simulink model "homing_ldm_aggiornat"  (R2017a)
settings: Solver=FixedStepAuto  StartTime=0.0  StopTime=inf  FixedStep=1e-3  RelTol=1e-3  EnableMultiTasking=on
values from neighbouring files (symbols this model uses):
  Acc_asse_x = []    [main_Strategia_di_pilotaggio.m]
  Acc_asse_y = []    [main_Strategia_di_pilotaggio.m]
  ppx_c = pos_poli_cc_x(mx, acx, 2)    [main_Strategia_di_pilotaggio.m]
  ppy_c = pos_poli_cc_y(my, acy, 2)    [main_Strategia_di_pilotaggio.m]
  time = 0:tf/np:tf    [Main_traiettoria.m]    (also in Main_traiettoria_ordinato.m = 0:passo:tsim)
  Vel_asse_x = []    [main_Strategia_di_pilotaggio.m]
  Vel_asse_y = []    [main_Strategia_di_pilotaggio.m]
  x = zeros(length(time),1)    [Main_traiettoria.m]    (also in Main_traiettoria_ordinato.m; main_Strategia_di_pilotaggio.m = [])
  y = zeros(length(time),1)    [Main_traiettoria.m]    (also in Main_traiettoria_ordinato.m; main_Strategia_di_pilotaggio.m = [])
undefined symbols (not defined in the file or in its folder): parx, pary, x_ref
libraries: xpcnilib x10, simulink x5
settings Model: SimulationMode=external  Creator=Davide  LastModifiedBy=stefa
settings SolverCC: EnableConcurrentExecution=on  ConcurrentTasks=on  AutoInsertRateTranBlk=on
settings DataIOCC: SaveFormat=StructureWithTime
settings OptimizationCC: BlockReduction=off  OptimizeBlockIOStorage=off  BufferReuse=off  GlobalBufferReuse=off  ExpressionFolding=off  LocalBlockOutputs=off
settings HardwareCC: ProdBitPerPointer=32  ProdBitPerSizeT=32  ProdBitPerPtrDiffT=32  ProdLargestAtomicFloat=None  ProdWordSize=32  ProdLongLongMode=on  ProdHWDeviceType=Generic->32-bit x86 compatible
settings RTWCC: SystemTargetFile=slrt.tlc  TemplateMakefile=slrt_default_tmf  Description=Simulink Real-Time  RTWCompilerOptimization=on
settings SimulinkRealTimeCC: xPCConcurrentTasks=on

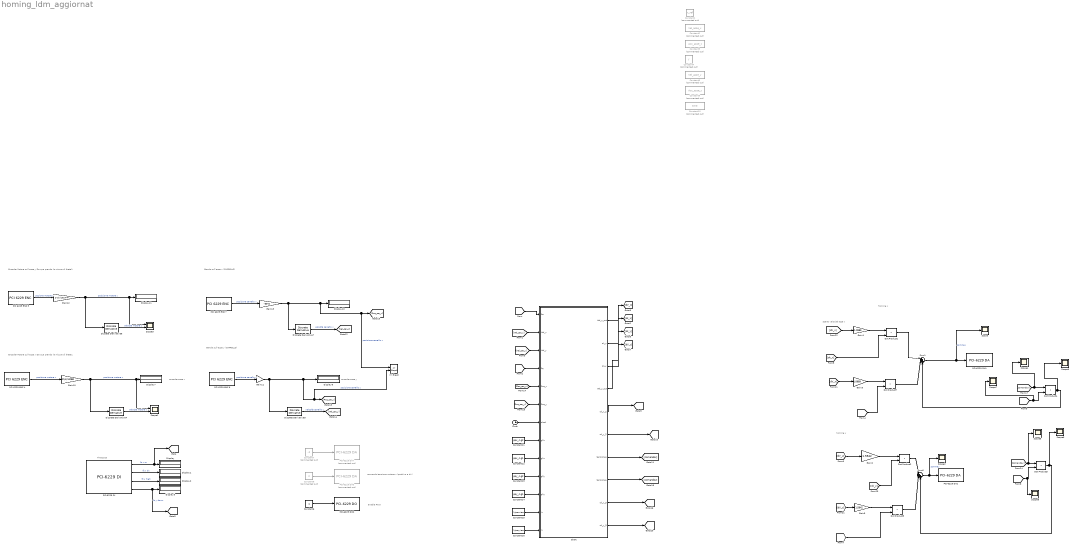
== system homing_ldm_aggiornat ==
  note: Finecorsa
  note: Encoder Motore sull'asse y
      | Da qua prendo la misura di theta1
  note: encoder asse y
  note: encoder asse x
  note: Banda sull'asse y (CARRELLO)
  note: comando tensione motore x (positivo a dx)
  note: Encoder Motore sull'asse x
      | Da qua prendo la misura di theta1
  note: enable P0.0
  note: Banda sull'asse x (CARRELLO)
  note: Scarto velocità asse x
  note: Homing x
  note: homing y
  Chart : Stateflow chart  TreatAsAtomicUnit=on
  Clock : Clock
  Constant1 : Constant  Commented=on  Value=x_ref
  Constant10 : Constant  Commented=on  Value=time
  Constant11 : Constant  Value=ppx_c.g2
  Constant12 : Constant  Value=ppx_c.g1
  Constant13 : Constant  Value=ppy_c.g2
  Constant14 : Constant  Value=ppy_c.g1
  Constant15 : Constant  Value=1/parx.tau
  Constant16 : Constant  Value=1/pary.tau
  Constant2 : Constant  Commented=on  Value=Vel_asse_x
  Constant3 : Constant  Commented=on  Value=Acc_asse_x
  Constant4 : Constant  Commented=on  Value=y
  Constant5 : Constant  Commented=on  Value=Vel_asse_y
  Constant6 : Constant
  Constant7 : Constant  Commented=on  Value=-2
  Constant8 : Constant  Commented=on  Value=2
  Constant9 : Constant  Commented=on  Value=Acc_asse_y
  Discrete Derivative{4..7} (4 alike) : simulink/Discrete/Discrete Derivative  gainval=1.0  ICPrevScaledInput=0.0  OutMin=[]  OutMax=[]  OutDataType=fixdt(1, 16)  OutScaling=2^-10  DoSatur=off
  Display{,1..3,7..8,10..11} (8 alike) : Display
  Dot Product{1..4,7..8} (6 alike) : DotProduct  InputSameDT=on  OutDataTypeStr=Inherit: Inherit via internal rule
  Gain1 : Gain  Gain=1.0989
  Gain10 : Gain  Gain=2*pi/(4096)
  Gain11 : Gain  Gain=-5e-6
  Gain12 : Gain  Gain=2*pi/(1024*4)
  Gain13 : Gain  Gain=-5e-6
  Gain2 : Gain  Gain=1.5942
  Gain3 : Gain  Gain=1.0989
  Gain5 : Gain  Gain=1.5942
  PCI 6229 ENC 4 : xpcnilib/Incremental Encoder/PCI 6229 ENC   channel=0  countMode=Quadrature Mode x4  initCount=0  reload=on  indexPhase=A low B low  filter=None  sampleTime=0.001  slot=[4 12]
      settings: SourceProductName=Simulink Real-Time  SourceProductBaseCode=XP
  PCI 6229 ENC 5 : xpcnilib/Incremental Encoder/PCI 6229 ENC   channel=1  countMode=Quadrature Mode x4  initCount=0  reload=on  indexPhase=A low B low  filter=None  sampleTime=0.001  slot=[4 12]
      settings: SourceProductName=Simulink Real-Time  SourceProductBaseCode=XP
  PCI 6229 ENC 6 : xpcnilib/Incremental Encoder/PCI 6229 ENC   channel=0  countMode=Quadrature Mode x4  initCount=0  reload=on  indexPhase=A low B low  filter=None  sampleTime=0.001  slot=[4 15]
      settings: SourceProductName=Simulink Real-Time  SourceProductBaseCode=XP
  PCI 6229 ENC 7 : xpcnilib/Incremental Encoder/PCI 6229 ENC   channel=1  countMode=Quadrature Mode x4  initCount=0  reload=on  indexPhase=A low B low  filter=None  sampleTime=0.001  slot=[4 15]
      settings: SourceProductName=Simulink Real-Time  SourceProductBaseCode=XP
  PCI-6229 DA1 : xpcnilib/D//A/M Series/PCI-6229 DA  channel=[1]  reset=[1]  initValue=[0]  sampletime=0.001  slot=[4 12]
      settings: SourceProductName=Simulink Real-Time  SourceProductBaseCode=XP
  PCI-6229 DA2 : xpcnilib/D//A/M Series/PCI-6229 DA  channel=[1]  reset=[1]  initValue=[0]  sampletime=0.001  slot=[4 15]
      settings: SourceProductName=Simulink Real-Time  SourceProductBaseCode=XP
  PCI-6229 DA6 : xpcnilib/D//A/M Series/PCI-6229 DA  Commented=on  channel=[1]  reset=[1]  initValue=[0]  sampletime=0.001  slot=[4 12]
      settings: SourceProductName=Simulink Real-Time  SourceProductBaseCode=XP
  PCI-6229 DA7 : xpcnilib/D//A/M Series/PCI-6229 DA  Commented=on  channel=[1]  reset=[1]  initValue=[0]  sampletime=0.001  slot=[4 15]
      settings: SourceProductName=Simulink Real-Time  SourceProductBaseCode=XP
  PCI-6229 DI : xpcnilib/Digital Input/M Series/PCI-6229 DI  channel=[4 5 6 7]  sampletime=0.001  slot=[4 12]
      settings: SourceProductName=Simulink Real-Time  SourceProductBaseCode=XP
  PCI-6229 DO2 : xpcnilib/Digital Output/M Series/PCI-6229 DO  channel=[1]  reset=[1]  initValue=[0]  sampletime=0.001  slot=[4 12]
      settings: SourceProductName=Simulink Real-Time  SourceProductBaseCode=XP
  Scope{,2,4..9} (8 alike) : Scope
  Scope1 : Scope  NumInputPorts=2
  Scope3 : Scope  NumInputPorts=2
  Sum1 : Sum  Inputs=|+++
  Sum6 : Sum  Inputs=|+++
  XY Graph : simulink/Sinks/XY Graph  xmin=-1  xmax=1  ymin=-1  ymax=1  st=-1
  wires:
  PCI-6229 DI/1 -> [Fcx_sx], Display/1  "fc x sx"
  PCI-6229 DI/2 -> Display1/1  "fc x dx"
  PCI-6229 DI/3 -> Display2/1  "fc y high"
  PCI-6229 DI/4 -> [Fcy_dw], Display3/1  "fc y down"
  [Fcx_sx] -> Chart/1(fcx)
  [Vel_car_x] -> Chart/2(Vel_x)
  Chart/1(Vel_x_out) -> [dV_x]
  [Fcy_dw] -> Chart/4(fcy)
  [Vel_car_y] -> Chart/3(Vel_y)
  Chart/2(ok_x) -> [ok_x]
  Chart/3(ok_y) -> [ok_y]
  Chart/4(Vel_y_out) -> [dV_y]
  [Pos_car_x] -> Chart/5(Pos_x)
  Chart/5(ok_x_2) -> [ok_x_2]
  Chart/6(ok_y_2) -> [ok_y_2]
  [Pos_car_y] -> Chart/6(Pos_y)
  Clock/1 -> Chart/7(clock)
  Gain13/1 -> Discrete Derivative7/1, XY Graph/1, [Pos_car_x], Display10/1  "posizione carrello x"
  Constant6/1 -> PCI-6229 DO2/1
  Constant8/1 -> PCI-6229 DA6/1
  Discrete Derivative4/1 -> Scope1/2  "velocità motore x"
  Discrete Derivative6/1 -> Scope3/2  "velocità motore y"
  Constant7/1 -> PCI-6229 DA7/1
  PCI 6229 ENC 5/1 -> Gain12/1  "pozione motore y"
  Discrete Derivative7/1 -> [Vel_car_x]  "velocità carrello x"
  Gain11/1 -> XY Graph/2, [Pos_car_y], Display8/1, Discrete Derivative5/1  "posizione carrello y"
  Gain10/1 -> Display7/1, Scope1/1, Discrete Derivative4/1  "posizione motore x"
  Discrete Derivative5/1 -> [Vel_car_y]  "velocità carrello y"
  PCI 6229 ENC 4/1 -> Gain10/1  "posizione motore x"
  PCI 6229 ENC 6/1 -> Gain11/1  "posizione carrello y"
  PCI 6229 ENC 7/1 -> Gain13/1  "posizione carrello x"
  Gain12/1 -> Scope3/1, Display11/1, Discrete Derivative6/1  "posizione motore y"
  Dot Product2/1 -> Sum6/1
  [dV_y] -> Gain5/1
  Gain3/1 -> Dot Product7/1
  Dot Product8/1 -> Sum6/2
  Sum6/1 -> Scope2/1, PCI-6229 DA2/1  "sommay"
  Sum1/1 -> Scope/1, PCI-6229 DA1/1  "sommax"
  Dot Product1/1 -> Sum1/1
  Gain5/1 -> Dot Product8/1
  Gain2/1 -> Dot Product2/1
  [ok_y_2] -> Dot Product8/2
  [ok_x_2] -> Dot Product7/2
  [dV_x] -> Gain3/1
  [ok_x] -> Dot Product1/2
  Dot Product7/1 -> Sum1/2
  Gain1/1 -> Dot Product1/1
  [dV_y] -> Gain2/1
  [dV_x] -> Gain1/1
  [ok_y] -> Dot Product2/2
  Constant11/1 -> Chart/8(g2x)
  Constant12/1 -> Chart/9(g1x)
  Constant13/1 -> Chart/10(g2y)
  Constant14/1 -> Chart/11(g1y)
  Constant15/1 -> Chart/12(ix)
  Constant16/1 -> Chart/13(iy)
  Chart/7(tensionex) -> [comandox]
  Chart/8(tensioney) -> [comandoy]
  Chart/10(ok_y_3) -> [ok_y_3]
  Chart/9(ok_x_3) -> [ok_x_3]
  Dot Product3/1 -> Scope6/1, Sum6/3
  [comandoy] -> Scope5/1, Dot Product3/1
  [ok_y_3] -> Scope8/1, Dot Product3/2
  Dot Product4/1 -> Scope9/1, Sum1/3
  [comandox] -> Scope4/1, Dot Product4/1
  [ok_x_3] -> Scope7/1, Dot Product4/2

== stateflow chart homing_ldm_aggiornat/Chart ==
  state Pilotaggio
    state Pilotaggio
      entry:
      t1=clock;
      ok_y_3=1;
      ok_x_3=1;
      deltax = 0;
      deltay = 0;
      deltaxp = 0;
      deltayp = 0;
      appoggio=1;
      rif_iniziale=0;
      during:
      t=clock-t1;
      if(clock-t1 ==0)
      rif_iniziale= t;
      end
      [rifx,rifxp,rify,rifyp]= interpolazione_tempi2(x, Vel_asse_x,y,Vel_asse_y,t,time,rif_iniziale)
      %[rifx,rifxp,rify,rifyp]= interpolazione_tempi2(x_i,xp_i,y_i,yp_i,u,t_m)
      deltax = Pos_x-rifx;
      deltay = Pos_y-rify;
      deltaxp = Vel_x-rifxp;
      deltayp = Vel_y-rifyp;
      %controllore posizionamento poli
      tensionex=ix*(-deltaxp*g2x-deltax*g1x)/30; %25
      tensioney=iy*(-deltayp*g2y-deltay*g1y)/50; %30
      if(tensioney>1.4)
      tensioney=1.4;
      end
      if(tensioney<-1.4)
      tensioney=-1.4;
      end
      if(tensionex>2.2)
      tensionex=2.2;
      end
      if(tensionex<-2.2)
      tensionex=-2.2;
      end
      %if tensionex ==0 && t<100
      % tensionex=2.1;
      % tensioney=0;
      % appoggio =0;
      %end
    state Fine
      entry:
      ok_y=0;
      ok_x=0;
      ok_y_2=0;
      ok_x_2=0;
      ok_y_3=0;
      ok_x_3=0;
    (default) -> Pilotaggio.Pilotaggio
    Pilotaggio.Pilotaggio -> Pilotaggio.Fine : [ abs(tensionex)==10 || abs(tensioney)==10]
  state Homing1
    state Homing_x
      entry:
      v_sp_x=-2.1;
      v_sp_y=1.2;
      ok_x=1;
      ok_y=1;
      ok_x_2=0;
      during:
      Vel_x_out = v_sp_x-Vel_x;
      Vel_y_out=v_sp_y-Vel_y;
    note: Inizializzazione asse x
        | Inizializzazione asse y
    state Fine_homing1
      entry:
      ok_y=0;
      ok_x=0;
      bx=Pos_x;
      by=Pos_y;
      v_sp_x=2.1;
      v_sp_y=-1.2;
      ok_x_2=1;
      ok_y_2=1;
      during:
      Vel_x_out=v_sp_x-Vel_x;
      dx=Pos_x-bx
      if (dx>0.6 )
      Vel_x_out=0;
      end
      Vel_y_out=v_sp_y-Vel_y;
      dy=abs(Pos_y-by);
      if (dy>0.4 )
      Vel_y_out=0;
      end
    note: Fine inizializzazione
    note: Porto al centro asse x
        | Porto al centro asse y
    state Fine
      entry:
      ok_y_2=0;
      ok_x_2=0;
      inizio_traiettoria=0;
      during:
      inizio_traiettoria=1;
    (default) -> Homing_x
    Homing_x -> Fine_homing1 : [fcx==0 && fcy==0]
    Fine_homing1 -> Homing1.Fine : [dx>0.6 && dy>0.4]
  (default) -> Homing1
  Homing1 -> Pilotaggio : [inizio_traiettoria==1]
  data: x_i function_input; xp_i function_input; y_i function_input; yp_i function_input; u function_input; t_m function_input; xx function_output; xxp function_output; yy function_output; yyp function_output; riff_iniziale function_input; t1 local double; t local double; fcx input; Vel_x_out output; Vel_x input; ok_x output; ok_y output; Vel_y input; Vel_y_out output; fcy input; Pos_x input; dx local; ok_x_2 output; v_sp_x local; v_sp_y local; Pos_y input; ok_y_2 output; dy local; clock input; bx local; by local; inizio_traiettoria local; g2x input; g1x input; g2y input; g1y input; deltaxp local; deltayp local; ix input; iy input; deltax local; deltay local; tensionex output; tensioney output; ok_x_3 output; ok_y_3 output; Vel_asse_x parameter; Vel_asse_y parameter; time parameter; x parameter; y parameter; rifx local; rifxp local; rify local; rifyp local; appoggio local; rif_iniziale local
  function [xx,xxp,yy,yyp]= interpolazione_tempi2(x_i,xp_i,y_i,yp_i,u,t_m,riff_iniziale):
    | function [xx,xxp,yy,yyp]= interpolazione_tempi2(x_i,xp_i,y_i,yp_i,u,t_m,riff_iniziale)
    | %interpolazione tempi asse x
    | xx= interp1(t_m,x_i,u,'Linear',riff_iniziale);
    | xxp= interp1(t_m,xp_i,u,'Linear',0);
    | 
    | %interpolazione tempi asse y
    | yy= interp1(t_m,y_i,u,'Linear',riff_iniziale);
    | yyp= interp1(t_m,yp_i,u,'Linear',0);
    | 
    | end
